simulink model "LLC_simscape3"  (R2022b)
settings: Solver=VariableStepAuto  StartTime=0.0  StopTime=0.01  MaxStep=1e-4  RelTol=1e-4
PreLoadFcn:
  | Rs_fet=1e8;  % FET snubber resistance (ohms)
  | Cs_fet=inf;  % FET snubber capacitance (ohms)
  | Vf=0.6;        % Diode forward voltage (V)
values from neighbouring files (symbols this model uses):
  Cr = 1/(2*pi*Rac_min*Qmax*fr)    (= 1.02444664021e-06)    [llc_verification.m]
  fr = 110e3    (= 110000)    [llc_verification.m]
  Lm = Lr*m-Lr    (= 1.08303232749e-05)    [llc_verification.m]
  Lr = Rac_min*Qmax/fr/2/pi    (= 2.04345722169e-06)    [llc_verification.m]
  n = Vin/Vo    (= 0.0825)    [llc_verification.m]
  Po = 250    [llc_verification.m]
  Vin = 33    [llc_verification.m]
libraries: spsDiodeLib x6, spsCurrentMeasurementLib x5, spsSeriesRLCBranchLib x4, spsIdealSwitchLib x4, spsVoltageMeasurementLib x4, spsOnDelayLib x2, spsControlledVoltageSourceLib x1, spsLinearTransformerLib x1, spspowerguiLib x1
settings Model: SimulationMode=accelerator  PauseTimes=0.001  Creator=Hyeongmeen Baik  LastModifiedBy=Hyeongmeen Baik
settings ModelReferenceCC: UpdateModelReferenceTargets=IfOutOfDate  EnableRefExpFcnMdlSchedulingChecks=on

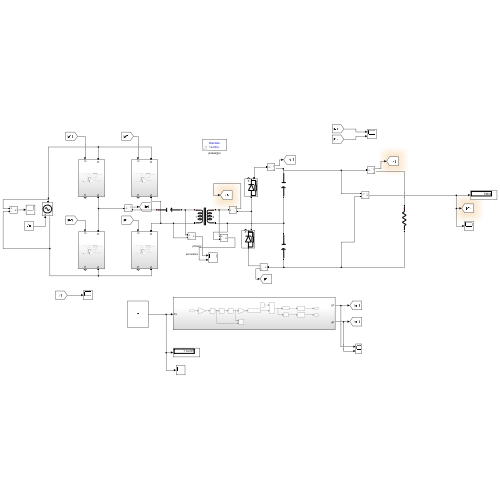
[thumbnail: Simulink's stored preview of the top-level diagram]
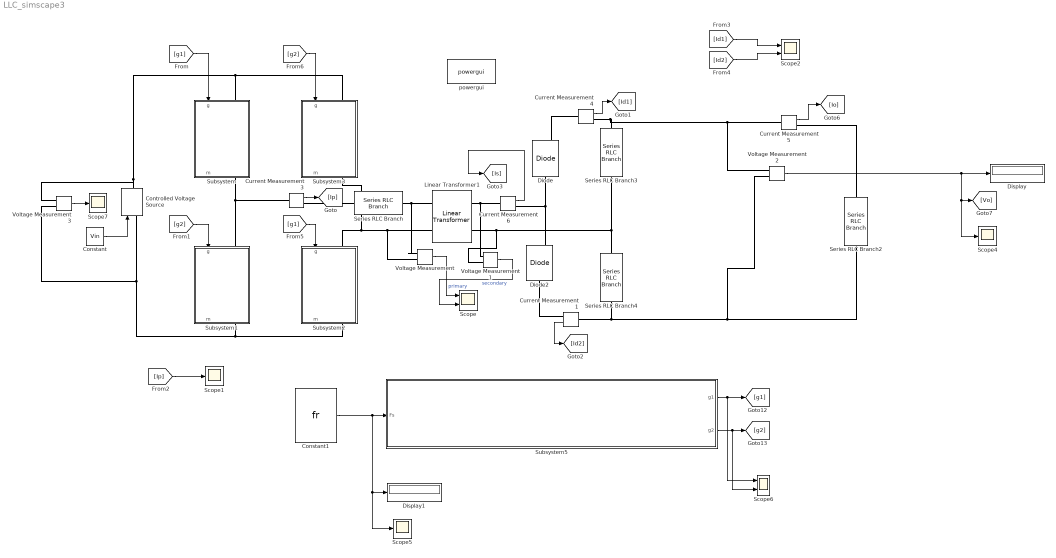
== system LLC_simscape3 ==
  Constant : Constant  Value=Vin
  Constant1 : Constant  Value=fr
  Controlled Voltage Source : spsControlledVoltageSourceLib/Controlled Voltage Source  Initialize=on  Source_Type=AC  Amplitude=0  Phase=0  Frequency=0  Measurements=None
  Current Measurement{1,3..6} (5 alike) : spsCurrentMeasurementLib/Current Measurement  PhasorSimulation=off  OutputType=Complex  PSBequivalent=0
  Diode : spsDiodeLib/Diode  Ron=1e-3  Lon=0  Vf=0.5  IC=0  UseSnubber=0  Rs=1e6  Cs=inf  Measurements=on
  Diode2 : spsDiodeLib/Diode  Ron=1e-3  Lon=0  Vf=0.5  IC=0  UseSnubber=0  Rs=1e6  Cs=inf  Measurements=on
  Display : Display
  Display1 : Display
  Linear Transformer1 : spsLinearTransformerLib/Linear Transformer  UNITS=SI  NominalPower=[ Po fr ]  winding1="[Vin   1e-2  Lr]"  winding2="[Vin/n  1e-2  Lr/100 ]"  ThreeWindings=off  winding3=[3.15e+05 9.9225e+05 74.316]  RmLm=[1e6 Lm]  Measurements=Magnetization current  DataType=on
  Scope : Scope  NumInputPorts=2
  Scope{1,4..5,7} (4 alike) : Scope
  Scope2 : Scope  NumInputPorts=2
  Scope6 : Scope  NumInputPorts=2
  Series RLC Branch : spsSeriesRLCBranchLib/Series RLC Branch  LConnTagsString=__new0  RConnTagsString=__new0  BranchType=C  Resistance=1  Inductance=1e-3  SetiL0=off  InitialCurrent=0  Capacitance=Cr  Setx0=off  InitialVoltage=0  Measurements=None
  Series RLC Branch2 : spsSeriesRLCBranchLib/Series RLC Branch  LConnTagsString=__new0  RConnTagsString=__new0  BranchType=R  Resistance=2560  Inductance=1e-3  SetiL0=off  InitialCurrent=0  Capacitance=1e-6  Setx0=off  InitialVoltage=0  Measurements=None
  Series RLC Branch3 : spsSeriesRLCBranchLib/Series RLC Branch  LConnTagsString=__new0  RConnTagsString=__new0  BranchType=C  Resistance=1  Inductance=1e-3  SetiL0=off  InitialCurrent=0  Capacitance=100e-6  Setx0=on  InitialVoltage=Vo  Measurements=None
  Series RLC Branch4 : spsSeriesRLCBranchLib/Series RLC Branch  LConnTagsString=__new0  RConnTagsString=__new0  BranchType=C  Resistance=1  Inductance=1e-3  SetiL0=off  InitialCurrent=0  Capacitance=100e-6  Setx0=on  InitialVoltage=Vo  Measurements=None
  Subsystem : Subsystem
  Subsystem1 : Subsystem
  Subsystem2 : Subsystem
  Subsystem3 : Subsystem
  Subsystem5 : Subsystem
  Voltage Measurement{,1..3} (4 alike) : spsVoltageMeasurementLib/Voltage Measurement  PhasorSimulation=off  OutputType=Complex  PSBequivalent=0
  powergui : spspowerguiLib/powergui  Priority=1  SimulationMode=Discrete  SampleTime=1e-8  frequency=60  Iterations=50  frequencyindice=0  Pbase=100e6  ErrMax=1e-4  UnitsV=kV  UnitsW=MW  buscounter=0  FunctionMessages=off  echomessages=off  EnableUseOfTLC=off  CurrentSourceSwitches=off  DisableSnubberDevices=off  DisableRonSwitches=off  DisableVfSwitches=off  DisplayEquations=off  AutomaticDiscreteSolvers=off  SolverType=Tustin/Backward Euler (TBE)  Interpol=off  ExternalGateDelay=off  methode=off  Ts=100  x0status=blocks  SPID=on  SwTol=0  HookPort=off  NonlinearTolerance=1e-4  nMaxIteration=100  ContinueOnMaxIteration=off  RestoreLinks=warning  ResistiveCurrentMeasurement=off  Frange=[0:2:500]  Ylog=off  Xlog=on  ShowGrid=off  save=off  variable=ZData  structure=0  ZoomFFT=off  StartTime=0.0  cycles=1  DisplayStyle=1  fundamental=60  FreqAxis=off  MaxFrequency=1000  frequencyindicesteady=1  RmsSteady=1  display=off
  wires:
  Voltage Measurement2/1 -> Scope4/1, [Vo], Display/1
  [g1] -> Subsystem2/1(g)
  Subsystem5/2(g2) -> Scope6/2, [g2]
  Constant1/1 -> Scope5/1, Display1/1, Subsystem5/1(Fs)
  Constant/1 -> Controlled Voltage Source/1
  Current Measurement5/1 -> [Io]
  [g2] -> Subsystem1/1(g)
  Current Measurement4/1 -> [Id1]
  Current Measurement6/1 -> [Is]
  [g1] -> Subsystem/1(g)
  Subsystem5/1(g1) -> Scope6/1, [g1]
  Voltage Measurement3/1 -> Scope7/1
  [g2] -> Subsystem3/1(g)
  Current Measurement3/1 -> [Ip]
  Voltage Measurement/1 -> Scope/1  "primary"
  Voltage Measurement1/1 -> Scope/2  "secondary"
  [Ip] -> Scope1/1
  [Id1] -> Scope2/1
  Current Measurement1/1 -> [Id2]
  [Id2] -> Scope2/2
  connections:
  Linear Transformer1/RConn2 -- Voltage Measurement1/LConn2 -- Series RLC Branch3/RConn1 -- Series RLC Branch4/LConn1
  Controlled Voltage Source/RConn1 -- Subsystem/LConn1 -- Subsystem3/LConn1 -- Voltage Measurement3/LConn1
  Series RLC Branch2/RConn1 -- Voltage Measurement2/LConn2 -- Current Measurement1/LConn1 -- Series RLC Branch4/RConn1
  Subsystem3/RConn1 -- Voltage Measurement/LConn2 -- Linear Transformer1/LConn2 -- Subsystem2/LConn1
  Controlled Voltage Source/LConn1 -- Subsystem1/RConn1 -- Subsystem2/RConn1 -- Voltage Measurement3/LConn2
  Current Measurement6/RConn1 -- Diode/LConn1 -- Diode2/RConn1
  Voltage Measurement2/LConn1 -- Current Measurement4/RConn1 -- Series RLC Branch3/LConn1 -- Current Measurement5/LConn1
  Current Measurement3/LConn1 -- Subsystem1/LConn1 -- Subsystem/RConn1
  Series RLC Branch/RConn1 -- Voltage Measurement/LConn1 -- Linear Transformer1/LConn1
  Series RLC Branch2/LConn1 -- Current Measurement5/RConn1
  Current Measurement6/LConn1 -- Voltage Measurement1/LConn1 -- Linear Transformer1/RConn1
  Series RLC Branch/LConn1 -- Current Measurement3/RConn1
  Diode/RConn1 -- Current Measurement4/LConn1
  Diode2/LConn1 -- Current Measurement1/RConn1

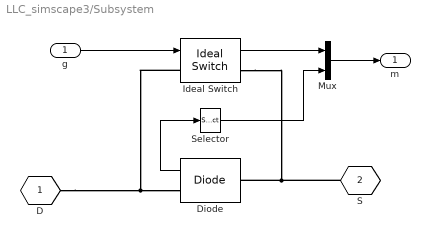
== system LLC_simscape3/Subsystem ==
  g : Inport
  Diode : spsDiodeLib/Diode  Ron=1e-3  Lon=0  Vf=Vf  IC=0  UseSnubber=0  Rs=inf  Cs=0  Measurements=on
  Ideal Switch : spsIdealSwitchLib/Ideal Switch  Ron=1e-3  Lon=0  IC=0  Rs=Rs_fet  Cs=Cs_fet  Measurements=on
  Mux : Mux  Inputs=[2,1]
  Selector : Selector  InputPortWidth=2  IndexOptions=Index vector (dialog)  Indices=1  OutputSizes=1
  D : PMIOPort  Tag=PMCPort  Side=Left
  S : PMIOPort  Tag=PMCPort  Port=2  Side=Right
  m : Outport  VectorParamsAs1DForOutWhenUnconnected=off
  wires:
  Ideal Switch/1 -> Mux/1
  Diode/1 -> Selector/1
  Mux/1 -> m/1
  g/1 -> Ideal Switch/1
  Selector/1 -> Mux/2
  connections:
  Ideal Switch/LConn1 -- Diode/RConn1 -- D/RConn1
  Ideal Switch/RConn1 -- Diode/LConn1 -- S/RConn1

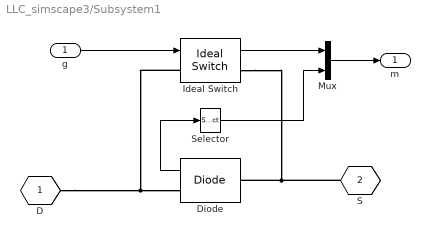
== system LLC_simscape3/Subsystem1 ==
  g : Inport
  Diode : spsDiodeLib/Diode  Ron=1e-3  Lon=0  Vf=Vf  IC=0  UseSnubber=0  Rs=inf  Cs=0  Measurements=on
  Ideal Switch : spsIdealSwitchLib/Ideal Switch  Ron=1e-3  Lon=0  IC=0  Rs=Rs_fet  Cs=Cs_fet  Measurements=on
  Mux : Mux  Inputs=[2,1]
  Selector : Selector  InputPortWidth=2  IndexOptions=Index vector (dialog)  Indices=1  OutputSizes=1
  D : PMIOPort  Tag=PMCPort  Side=Left
  S : PMIOPort  Tag=PMCPort  Port=2  Side=Right
  m : Outport  VectorParamsAs1DForOutWhenUnconnected=off
  wires:
  Ideal Switch/1 -> Mux/1
  Diode/1 -> Selector/1
  Mux/1 -> m/1
  g/1 -> Ideal Switch/1
  Selector/1 -> Mux/2
  connections:
  Ideal Switch/LConn1 -- Diode/RConn1 -- D/RConn1
  Ideal Switch/RConn1 -- Diode/LConn1 -- S/RConn1

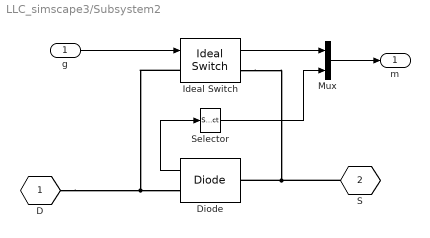
== system LLC_simscape3/Subsystem2 ==
  g : Inport
  Diode : spsDiodeLib/Diode  Ron=1e-3  Lon=0  Vf=Vf  IC=0  UseSnubber=0  Rs=inf  Cs=0  Measurements=on
  Ideal Switch : spsIdealSwitchLib/Ideal Switch  Ron=1e-3  Lon=0  IC=0  Rs=Rs_fet  Cs=Cs_fet  Measurements=on
  Mux : Mux  Inputs=[2,1]
  Selector : Selector  InputPortWidth=2  IndexOptions=Index vector (dialog)  Indices=1  OutputSizes=1
  D : PMIOPort  Tag=PMCPort  Side=Left
  S : PMIOPort  Tag=PMCPort  Port=2  Side=Right
  m : Outport  VectorParamsAs1DForOutWhenUnconnected=off
  wires:
  Ideal Switch/1 -> Mux/1
  Diode/1 -> Selector/1
  Mux/1 -> m/1
  g/1 -> Ideal Switch/1
  Selector/1 -> Mux/2
  connections:
  Ideal Switch/LConn1 -- Diode/RConn1 -- D/RConn1
  Ideal Switch/RConn1 -- Diode/LConn1 -- S/RConn1

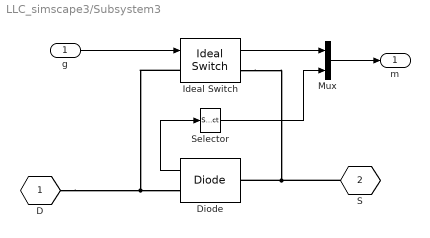
== system LLC_simscape3/Subsystem3 ==
  g : Inport
  Diode : spsDiodeLib/Diode  Ron=1e-3  Lon=0  Vf=Vf  IC=0  UseSnubber=0  Rs=inf  Cs=0  Measurements=on
  Ideal Switch : spsIdealSwitchLib/Ideal Switch  Ron=1e-3  Lon=0  IC=0  Rs=Rs_fet  Cs=Cs_fet  Measurements=on
  Mux : Mux  Inputs=[2,1]
  Selector : Selector  InputPortWidth=2  IndexOptions=Index vector (dialog)  Indices=1  OutputSizes=1
  D : PMIOPort  Tag=PMCPort  Side=Left
  S : PMIOPort  Tag=PMCPort  Port=2  Side=Right
  m : Outport  VectorParamsAs1DForOutWhenUnconnected=off
  wires:
  Ideal Switch/1 -> Mux/1
  Diode/1 -> Selector/1
  Mux/1 -> m/1
  g/1 -> Ideal Switch/1
  Selector/1 -> Mux/2
  connections:
  Ideal Switch/LConn1 -- Diode/RConn1 -- D/RConn1
  Ideal Switch/RConn1 -- Diode/LConn1 -- S/RConn1

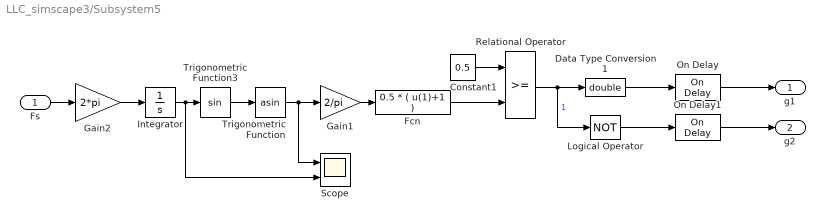
== system LLC_simscape3/Subsystem5 ==
  Fs : Inport
  Constant1 : Constant  Value=0.5
  Data Type Conversion1 : DataTypeConversion  OutDataTypeStr=double  SaturateOnIntegerOverflow=off  RndMeth=Floor
  Fcn : Fcn  Expr=0.5 * ( u(1)+1 )
  Gain1 : Gain  Gain=2/pi  SaturateOnIntegerOverflow=on  OutDataTypeStr=Inherit: Same as input  ParamDataTypeStr=Inherit: Same as input
  Gain2 : Gain  Gain=2*pi  SaturateOnIntegerOverflow=on  OutDataTypeStr=Inherit: Same as input  ParamDataTypeStr=Inherit: Same as input
  Integrator : Integrator
  Logical Operator : Logic  Operator=NOT  AllPortsSameDT=off  OutDataTypeStr=float('double')
  On Delay : spsOnDelayLib/On Delay  DelayType=On delay  delay=400e-9  ic=0  Ts=0
  On Delay1 : spsOnDelayLib/On Delay  DelayType=On delay  delay=400e-9  ic=0  Ts=0
  Relational Operator : RelationalOperator  OutDataTypeStr=boolean  InputSameDT=off
  Scope : Scope  NumInputPorts=2
  Trigonometric Function : Trigonometry  Operator=asin
  Trigonometric Function3 : Trigonometry
  g1 : Outport
  g2 : Outport  Port=2
  wires:
  Fs/1 -> Gain2/1
  Integrator/1 -> Scope/2, Trigonometric Function3/1
  On Delay1/1 -> g2/1
  Trigonometric Function3/1 -> Trigonometric Function/1
  Fcn/1 -> Relational Operator/2
  Logical Operator/1 -> On Delay1/1
  Trigonometric Function/1 -> Gain1/1, Scope/1
  Data Type Conversion1/1 -> On Delay/1
  On Delay/1 -> g1/1
  Constant1/1 -> Relational Operator/1
  Relational Operator/1 -> Data Type Conversion1/1, Logical Operator/1  "1"
  Gain2/1 -> Integrator/1
  Gain1/1 -> Fcn/1
